simulink library "BTM_lib"  (Simulink 7.4)
settings: Solver=ode45  StartTime=0.0  StopTime=10.0  RelTol=1e-3
values from neighbouring files (symbols this model uses):
  BTMc_t_AirOutMaxTemp_fault = mpt.Parameter    [BTM_CAL.m]
  BTMc_t_AirOutMaxTemp_warn = mpt.Parameter    [BTM_CAL.m]
  BTMc_t_BCUTempOver_fatal = mpt.Parameter    [BTM_CAL.m]
  BTMc_t_BCUTempOver_fault = mpt.Parameter    [BTM_CAL.m]
  BTMc_t_BCUTempOver_warn = mpt.Parameter    [BTM_CAL.m]
  BTMc_t_BMUTempOver_fatal = mpt.Parameter    [BTM_CAL.m]
  BTMc_t_BMUTempOver_fault = mpt.Parameter    [BTM_CAL.m]
  BTMc_t_BMUTempOver_warn = mpt.Parameter    [BTM_CAL.m]
  BTMc_t_MdlTempDifOver_fatal = mpt.Parameter    [BTM_CAL.m]
  BTMc_t_MdlTempDifOver_fault = mpt.Parameter    [BTM_CAL.m]
  BTMc_t_MdlTempDifOver_warn = mpt.Parameter    [BTM_CAL.m]
  BTMc_t_MdlTempOver_fatal = mpt.Parameter    [BTM_CAL.m]
  BTMc_t_MdlTempOver_fault = mpt.Parameter    [BTM_CAL.m]
  BTMc_t_MdlTempOver_warn = mpt.Parameter    [BTM_CAL.m]
  BTMc_t_MdlTempUnder_fatal = mpt.Parameter    [BTM_CAL.m]
  BTMc_t_MdlTempUnder_fault = mpt.Parameter    [BTM_CAL.m]
  BTMc_t_MdlTempUnder_warn = mpt.Parameter    [BTM_CAL.m]
undefined symbols (not defined in the file or in its folder): PACK_Const_MdlNumOfPack, PACK_Const_TempSnrNumOfMdl
settings Model: Creator=zhangyunyun  LastModifiedBy=sunsijun

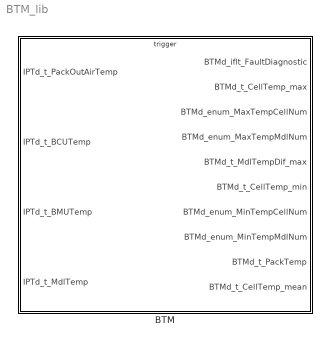
== system BTM_lib ==
  BTM : Subsystem  TreatAsAtomicUnit=on

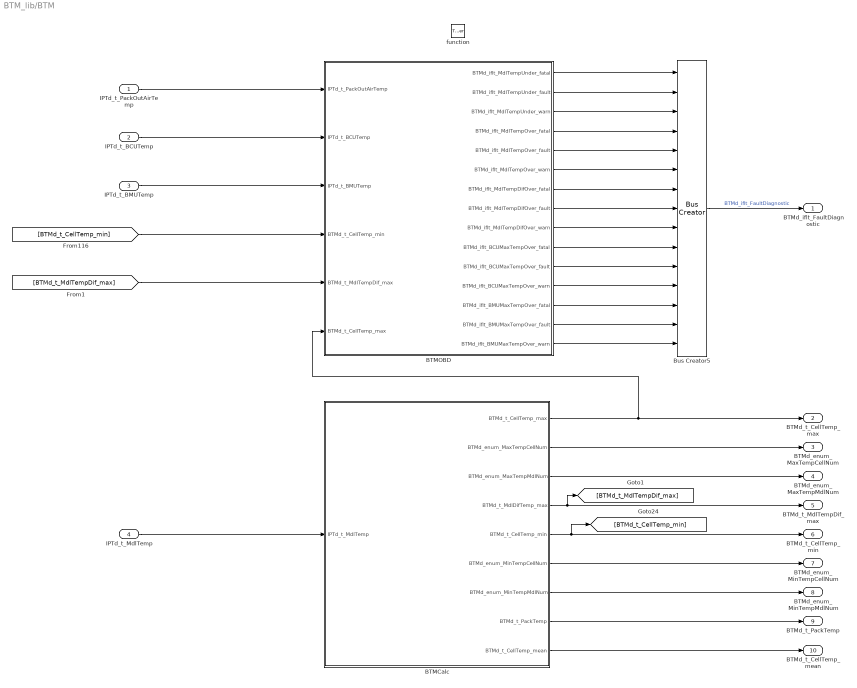
== system BTM_lib/BTM ==
  IPTd_t_PackOutAirTemp : Inport
  IPTd_t_BCUTemp : Inport  Port=2
  IPTd_t_BMUTemp : Inport  Port=3
  IPTd_t_MdlTemp : Inport  Port=4  DataType=single  OutDataTypeStr=single
  function : TriggerPort  TriggerType=function-call
  BTMCalc : Subsystem
  BTMOBD : Subsystem
  Bus Creator5 : BusCreator  Inputs=15
  BTMd_iflt_FaultDiagnostic : Outport  OutDataType=fixdt(1, 16)  OutScaling=2^0
  BTMd_t_CellTemp_max : Outport  Port=2  OutDataType=fixdt(1, 16)  OutScaling=2^0
  BTMd_enum_MaxTempCellNum : Outport  Port=3  OutDataType=fixdt(1, 16)  OutScaling=2^0
  BTMd_enum_MaxTempMdlNum : Outport  Port=4  OutDataType=fixdt(1, 16)  OutScaling=2^0
  BTMd_t_MdlTempDif_max : Outport  Port=5  OutDataType=fixdt(1, 16)  OutScaling=2^0
  BTMd_t_CellTemp_min : Outport  Port=6  OutDataType=fixdt(1, 16)  OutScaling=2^0
  BTMd_enum_MinTempCellNum : Outport  Port=7  OutDataType=fixdt(1, 16)  OutScaling=2^0
  BTMd_enum_MinTempMdlNum : Outport  Port=8  OutDataType=fixdt(1, 16)  OutScaling=2^0
  BTMd_t_PackTemp : Outport  Port=9  OutDataType=fixdt(1, 16)  OutScaling=2^0
  BTMd_t_CellTemp_mean : Outport  Port=10  OutDataType=fixdt(1, 16)  OutScaling=2^0
  wires:
  [BTMd_t_MdlTempDif_max] -> BTMOBD/5(BTMd_t_MdlTempDif_max)
  [BTMd_t_CellTemp_min] -> BTMOBD/4(BTMd_t_CellTemp_min)
  IPTd_t_BMUTemp/1 -> BTMOBD/3(IPTd_t_BMUTemp)
  BTMCalc/7(BTMd_enum_MinTempMdlNum) -> BTMd_enum_MinTempMdlNum/1
  BTMCalc/9(BTMd_t_CellTemp_mean) -> BTMd_t_CellTemp_mean/1
  BTMCalc/3(BTMd_enum_MaxTempMdlNum) -> BTMd_enum_MaxTempMdlNum/1
  IPTd_t_BCUTemp/1 -> BTMOBD/2(IPTd_t_BCUTemp)
  IPTd_t_PackOutAirTemp/1 -> BTMOBD/1(IPTd_t_PackOutAirTemp)
  BTMCalc/6(BTMd_enum_MinTempCellNum) -> BTMd_enum_MinTempCellNum/1
  IPTd_t_MdlTemp/1 -> BTMCalc/1(IPTd_t_MdlTemp)
  BTMCalc/4(BTMd_t_MdlDifTemp_max) -> [BTMd_t_MdlTempDif_max], BTMd_t_MdlTempDif_max/1
  BTMCalc/5(BTMd_t_CellTemp_min) -> [BTMd_t_CellTemp_min], BTMd_t_CellTemp_min/1
  BTMCalc/8(BTMd_t_PackTemp) -> BTMd_t_PackTemp/1
  BTMCalc/2(BTMd_enum_MaxTempCellNum) -> BTMd_enum_MaxTempCellNum/1
  BTMCalc/1(BTMd_t_CellTemp_max) -> BTMOBD/6(BTMd_t_CellTemp_max), BTMd_t_CellTemp_max/1
  BTMOBD/1(BTMd_iflt_MdlTempUnder_fatal) -> Bus Creator5/1
  BTMOBD/2(BTMd_iflt_MdlTempUnder_fault) -> Bus Creator5/2
  BTMOBD/3(BTMd_iflt_MdlTempUnder_warn) -> Bus Creator5/3
  BTMOBD/4(BTMd_iflt_MdlTempOver_fatal) -> Bus Creator5/4
  BTMOBD/5(BTMd_iflt_MdlTempOver_fault) -> Bus Creator5/5
  BTMOBD/6(BTMd_iflt_MdlTempOver_warn) -> Bus Creator5/6
  BTMOBD/7(BTMd_iflt_MdlTempDifOver_fatal) -> Bus Creator5/7
  BTMOBD/8(BTMd_iflt_MdlTempDifOver_fault) -> Bus Creator5/8
  BTMOBD/9(BTMd_iflt_MdlTempDifOver_warn) -> Bus Creator5/9
  BTMOBD/10(BTMd_iflt_BCUMaxTempOver_fatal) -> Bus Creator5/10
  BTMOBD/11(BTMd_iflt_BCUMaxTempOver_fault) -> Bus Creator5/11
  BTMOBD/12(BTMd_iflt_BCUMaxTempOver_warn) -> Bus Creator5/12
  BTMOBD/13(BTMd_iflt_BMUMaxTempOver_fatal) -> Bus Creator5/13
  BTMOBD/14(BTMd_iflt_BMUMaxTempOver_fault) -> Bus Creator5/14
  BTMOBD/15(BTMd_iflt_BMUMaxTempOver_warn) -> Bus Creator5/15
  Bus Creator5/1 -> BTMd_iflt_FaultDiagnostic/1  "BTMd_iflt_FaultDiagnostic"

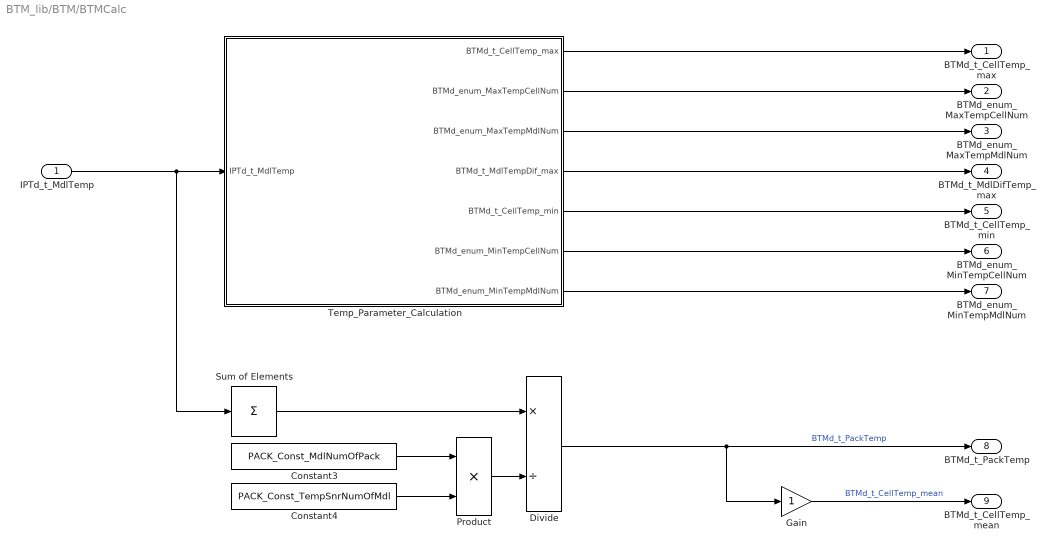
== system BTM_lib/BTM/BTMCalc ==
  IPTd_t_MdlTemp : Inport
  Constant3 : Constant  Value=PACK_Const_MdlNumOfPack  OutDataTypeMode=uint16  OutDataType=fixdt(1, 16)  OutScaling=2^0  OutDataTypeStr=uint16
  Constant4 : Constant  Value=PACK_Const_TempSnrNumOfMdl  OutDataTypeMode=uint16  OutDataType=fixdt(1, 16)  OutScaling=2^0  OutDataTypeStr=uint16
  Divide : Product  Inputs=*/  OutDataType=fixdt(1, 16)  OutScaling=2^-10
  Gain : Gain  ParameterDataType=fixdt(1, 16)  ParameterScaling=2^0  OutDataType=fixdt(1, 16)  OutScaling=2^0
  Product : Product  OutDataType=fixdt(1, 16)  OutScaling=2^0  RndMeth=Zero
  Sum of Elements : Sum  Inputs=+  OutDataType=fixdt(1, 16)  OutScaling=2^-10
  Temp_Parameter_Calculation : Subsystem  TreatAsAtomicUnit=on
  BTMd_t_CellTemp_max : Outport  OutDataType=fixdt(1, 16)  OutScaling=2^0
  BTMd_enum_MaxTempCellNum : Outport  Port=2  OutDataType=fixdt(1, 16)  OutScaling=2^0
  BTMd_enum_MaxTempMdlNum : Outport  Port=3  OutDataType=fixdt(1, 16)  OutScaling=2^0
  BTMd_t_MdlDifTemp_max : Outport  Port=4  OutDataType=fixdt(1, 16)  OutScaling=2^0
  BTMd_t_CellTemp_min : Outport  Port=5  OutDataType=fixdt(1, 16)  OutScaling=2^0
  BTMd_enum_MinTempCellNum : Outport  Port=6  OutDataType=fixdt(1, 16)  OutScaling=2^0
  BTMd_enum_MinTempMdlNum : Outport  Port=7  OutDataType=fixdt(1, 16)  OutScaling=2^0
  BTMd_t_PackTemp : Outport  Port=8
  BTMd_t_CellTemp_mean : Outport  Port=9  OutDataType=fixdt(1, 16)  OutScaling=2^0
  wires:
  Temp_Parameter_Calculation/7(BTMd_enum_MinTempMdlNum) -> BTMd_enum_MinTempMdlNum/1
  Gain/1 -> BTMd_t_CellTemp_mean/1  "BTMd_t_CellTemp_mean"
  Temp_Parameter_Calculation/3(BTMd_enum_MaxTempMdlNum) -> BTMd_enum_MaxTempMdlNum/1
  Temp_Parameter_Calculation/6(BTMd_enum_MinTempCellNum) -> BTMd_enum_MinTempCellNum/1
  Product/1 -> Divide/2
  Sum of Elements/1 -> Divide/1
  Temp_Parameter_Calculation/4(BTMd_t_MdlTempDif_max) -> BTMd_t_MdlDifTemp_max/1
  Temp_Parameter_Calculation/5(BTMd_t_CellTemp_min) -> BTMd_t_CellTemp_min/1
  Temp_Parameter_Calculation/1(BTMd_t_CellTemp_max) -> BTMd_t_CellTemp_max/1
  Divide/1 -> Gain/1, BTMd_t_PackTemp/1  "BTMd_t_PackTemp"
  IPTd_t_MdlTemp/1 -> Sum of Elements/1, Temp_Parameter_Calculation/1(IPTd_t_MdlTemp)
  Temp_Parameter_Calculation/2(BTMd_enum_MaxTempCellNum) -> BTMd_enum_MaxTempCellNum/1
  Constant3/1 -> Product/1
  Constant4/1 -> Product/2

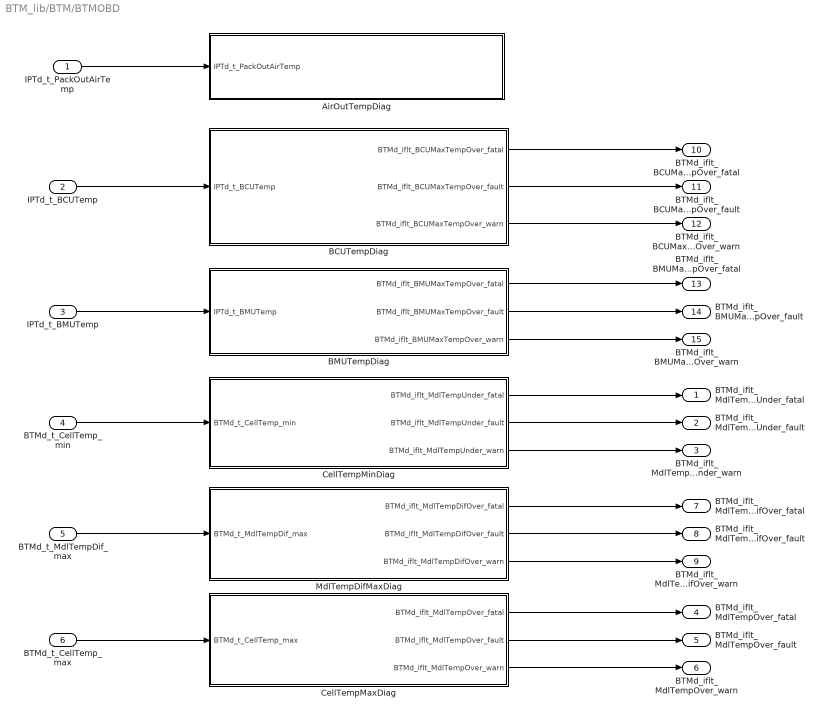
== system BTM_lib/BTM/BTMOBD ==
  IPTd_t_PackOutAirTemp : Inport
  IPTd_t_BCUTemp : Inport  Port=2
  IPTd_t_BMUTemp : Inport  Port=3
  BTMd_t_CellTemp_min : Inport  Port=4  OutDataType=fixdt(1, 16)  OutScaling=2^0
  BTMd_t_MdlTempDif_max : Inport  Port=5  OutDataType=fixdt(1, 16)  OutScaling=2^0
  BTMd_t_CellTemp_max : Inport  Port=6  OutDataType=fixdt(1, 16)  OutScaling=2^0
  AirOutTempDiag : Subsystem  TreatAsAtomicUnit=on
  BCUTempDiag : Subsystem  TreatAsAtomicUnit=on
  BMUTempDiag : Subsystem  TreatAsAtomicUnit=on
  CellTempMaxDiag : Subsystem  TreatAsAtomicUnit=on
  CellTempMinDiag : Subsystem  TreatAsAtomicUnit=on
  MdlTempDifMaxDiag : Subsystem  TreatAsAtomicUnit=on
  BTMd_iflt_MdlTempUnder_fatal : Outport  OutDataType=fixdt(1, 16)  OutScaling=2^0
  BTMd_iflt_MdlTempUnder_fault : Outport  Port=2  OutDataType=fixdt(1, 16)  OutScaling=2^0
  BTMd_iflt_MdlTempUnder_warn : Outport  Port=3  OutDataType=fixdt(1, 16)  OutScaling=2^0
  BTMd_iflt_MdlTempOver_fatal : Outport  Port=4  OutDataType=fixdt(1, 16)  OutScaling=2^0
  BTMd_iflt_MdlTempOver_fault : Outport  Port=5  OutDataType=fixdt(1, 16)  OutScaling=2^0
  BTMd_iflt_MdlTempOver_warn : Outport  Port=6  OutDataType=fixdt(1, 16)  OutScaling=2^0
  BTMd_iflt_MdlTempDifOver_fatal : Outport  Port=7  OutDataType=fixdt(1, 16)  OutScaling=2^0
  BTMd_iflt_MdlTempDifOver_fault : Outport  Port=8  OutDataType=fixdt(1, 16)  OutScaling=2^0
  BTMd_iflt_MdlTempDifOver_warn : Outport  Port=9  OutDataType=fixdt(1, 16)  OutScaling=2^0
  BTMd_iflt_BCUMaxTempOver_fatal : Outport  Port=10  OutDataType=fixdt(1, 16)  OutScaling=2^0
  BTMd_iflt_BCUMaxTempOver_fault : Outport  Port=11  OutDataType=fixdt(1, 16)  OutScaling=2^0
  BTMd_iflt_BCUMaxTempOver_warn : Outport  Port=12  OutDataType=fixdt(1, 16)  OutScaling=2^0
  BTMd_iflt_BMUMaxTempOver_fatal : Outport  Port=13  OutDataType=fixdt(1, 16)  OutScaling=2^0
  BTMd_iflt_BMUMaxTempOver_fault : Outport  Port=14  OutDataType=fixdt(1, 16)  OutScaling=2^0
  BTMd_iflt_BMUMaxTempOver_warn : Outport  Port=15  OutDataType=fixdt(1, 16)  OutScaling=2^0
  wires:
  MdlTempDifMaxDiag/3(BTMd_iflt_MdlTempDifOver_warn) -> BTMd_iflt_MdlTempDifOver_warn/1
  MdlTempDifMaxDiag/2(BTMd_iflt_MdlTempDifOver_fault) -> BTMd_iflt_MdlTempDifOver_fault/1
  MdlTempDifMaxDiag/1(BTMd_iflt_MdlTempDifOver_fatal) -> BTMd_iflt_MdlTempDifOver_fatal/1
  BTMd_t_MdlTempDif_max/1 -> MdlTempDifMaxDiag/1(BTMd_t_MdlTempDif_max)
  CellTempMaxDiag/3(BTMd_iflt_MdlTempOver_warn) -> BTMd_iflt_MdlTempOver_warn/1
  CellTempMaxDiag/2(BTMd_iflt_MdlTempOver_fault) -> BTMd_iflt_MdlTempOver_fault/1
  CellTempMaxDiag/1(BTMd_iflt_MdlTempOver_fatal) -> BTMd_iflt_MdlTempOver_fatal/1
  BTMd_t_CellTemp_max/1 -> CellTempMaxDiag/1(BTMd_t_CellTemp_max)
  CellTempMinDiag/3(BTMd_iflt_MdlTempUnder_warn) -> BTMd_iflt_MdlTempUnder_warn/1
  CellTempMinDiag/2(BTMd_iflt_MdlTempUnder_fault) -> BTMd_iflt_MdlTempUnder_fault/1
  CellTempMinDiag/1(BTMd_iflt_MdlTempUnder_fatal) -> BTMd_iflt_MdlTempUnder_fatal/1
  BTMd_t_CellTemp_min/1 -> CellTempMinDiag/1(BTMd_t_CellTemp_min)
  BMUTempDiag/3(BTMd_iflt_BMUMaxTempOver_warn) -> BTMd_iflt_BMUMaxTempOver_warn/1
  BMUTempDiag/2(BTMd_iflt_BMUMaxTempOver_fault) -> BTMd_iflt_BMUMaxTempOver_fault/1
  BMUTempDiag/1(BTMd_iflt_BMUMaxTempOver_fatal) -> BTMd_iflt_BMUMaxTempOver_fatal/1
  IPTd_t_BMUTemp/1 -> BMUTempDiag/1(IPTd_t_BMUTemp)
  BCUTempDiag/3(BTMd_iflt_BCUMaxTempOver_warn) -> BTMd_iflt_BCUMaxTempOver_warn/1
  BCUTempDiag/2(BTMd_iflt_BCUMaxTempOver_fault) -> BTMd_iflt_BCUMaxTempOver_fault/1
  BCUTempDiag/1(BTMd_iflt_BCUMaxTempOver_fatal) -> BTMd_iflt_BCUMaxTempOver_fatal/1
  IPTd_t_BCUTemp/1 -> BCUTempDiag/1(IPTd_t_BCUTemp)
  IPTd_t_PackOutAirTemp/1 -> AirOutTempDiag/1(IPTd_t_PackOutAirTemp)

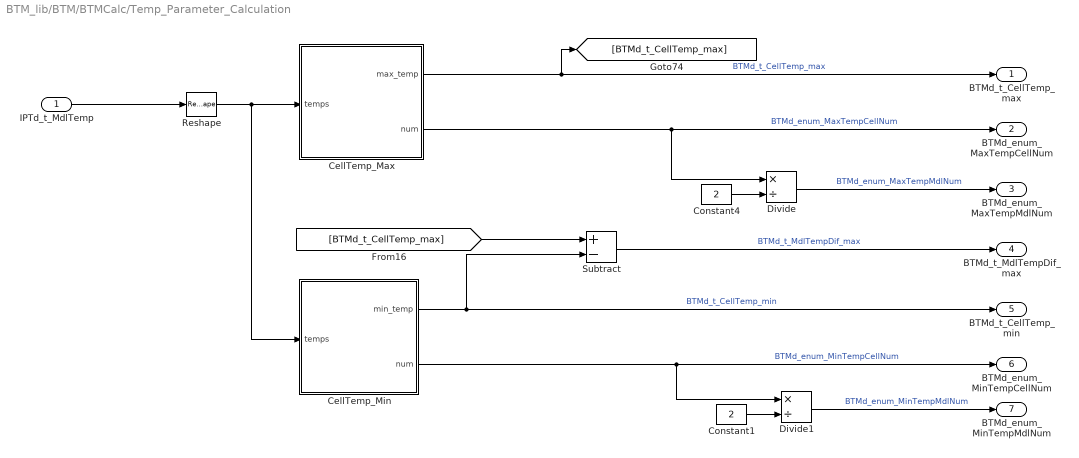
== system BTM_lib/BTM/BTMCalc/Temp_Parameter_Calculation ==
  IPTd_t_MdlTemp : Inport  OutDataType=fixdt(1, 16)  OutScaling=2^0
  CellTemp_Max : Stateflow chart
  CellTemp_Min : Stateflow chart
  Constant1 : Constant  Value=2  OutDataTypeMode=uint8  OutDataType=fixdt(1, 16)  OutScaling=2^0  OutDataTypeStr=uint8
  Constant4 : Constant  Value=2  OutDataTypeMode=uint8  OutDataType=fixdt(1, 16)  OutScaling=2^0  OutDataTypeStr=uint8
  Divide : Product  Inputs=*/  OutDataTypeMode=uint8  OutDataType=fixdt(1, 16)  OutScaling=2^-10  OutDataTypeStr=uint8  RndMeth=Ceiling
  Divide1 : Product  Inputs=*/  OutDataTypeMode=uint8  OutDataType=fixdt(1, 16)  OutScaling=2^-10  OutDataTypeStr=uint8  RndMeth=Ceiling
  Reshape : Reshape
  Subtract : Sum  Inputs=+-  OutDataType=fixdt(1, 16)  OutScaling=2^-10
  BTMd_t_CellTemp_max : Outport  OutDataType=fixdt(1, 16)  OutScaling=2^0
  BTMd_enum_MaxTempCellNum : Outport  Port=2  OutDataType=fixdt(1, 16)  OutScaling=2^0
  BTMd_enum_MaxTempMdlNum : Outport  Port=3  OutDataType=fixdt(1, 16)  OutScaling=2^0
  BTMd_t_MdlTempDif_max : Outport  Port=4  OutDataType=fixdt(1, 16)  OutScaling=2^0
  BTMd_t_CellTemp_min : Outport  Port=5  OutDataType=fixdt(1, 16)  OutScaling=2^0
  BTMd_enum_MinTempCellNum : Outport  Port=6  OutDataType=fixdt(1, 16)  OutScaling=2^0
  BTMd_enum_MinTempMdlNum : Outport  Port=7  OutDataType=fixdt(1, 16)  OutScaling=2^0
  wires:
  [BTMd_t_CellTemp_max] -> Subtract/1
  Divide1/1 -> BTMd_enum_MinTempMdlNum/1  "BTMd_enum_MinTempMdlNum"
  Constant1/1 -> Divide1/2
  Divide/1 -> BTMd_enum_MaxTempMdlNum/1  "BTMd_enum_MaxTempMdlNum"
  Constant4/1 -> Divide/2
  CellTemp_Min/2(num) -> Divide1/1, BTMd_enum_MinTempCellNum/1  "BTMd_enum_MinTempCellNum"
  Subtract/1 -> BTMd_t_MdlTempDif_max/1  "BTMd_t_MdlTempDif_max"
  CellTemp_Min/1(min_temp) -> Subtract/2, BTMd_t_CellTemp_min/1  "BTMd_t_CellTemp_min"
  Reshape/1 -> CellTemp_Min/1(temps), CellTemp_Max/1(temps)
  IPTd_t_MdlTemp/1 -> Reshape/1
  CellTemp_Max/2(num) -> Divide/1, BTMd_enum_MaxTempCellNum/1  "BTMd_enum_MaxTempCellNum"
  CellTemp_Max/1(max_temp) -> BTMd_t_CellTemp_max/1, [BTMd_t_CellTemp_max]  "BTMd_t_CellTemp_max"

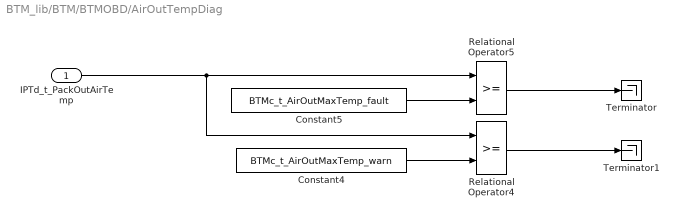
== system BTM_lib/BTM/BTMOBD/AirOutTempDiag ==
  IPTd_t_PackOutAirTemp : Inport
  Constant4 : Constant  Value=BTMc_t_AirOutMaxTemp_warn  OutDataType=fixdt(1, 16)  OutScaling=2^0
  Constant5 : Constant  Value=BTMc_t_AirOutMaxTemp_fault  OutDataType=fixdt(1, 16)  OutScaling=2^0
  Relational Operator4 : RelationalOperator  LogicOutDataTypeMode=boolean  LogicDataType=fixdt(0, 8)  OutDataTypeStr=boolean
  Relational Operator5 : RelationalOperator  LogicOutDataTypeMode=boolean  LogicDataType=fixdt(0, 8)  OutDataTypeStr=boolean
  Terminator : Terminator
  Terminator1 : Terminator
  wires:
  IPTd_t_PackOutAirTemp/1 -> Relational Operator5/1, Relational Operator4/1
  Constant5/1 -> Relational Operator5/2
  Constant4/1 -> Relational Operator4/2
  Relational Operator4/1 -> Terminator1/1
  Relational Operator5/1 -> Terminator/1

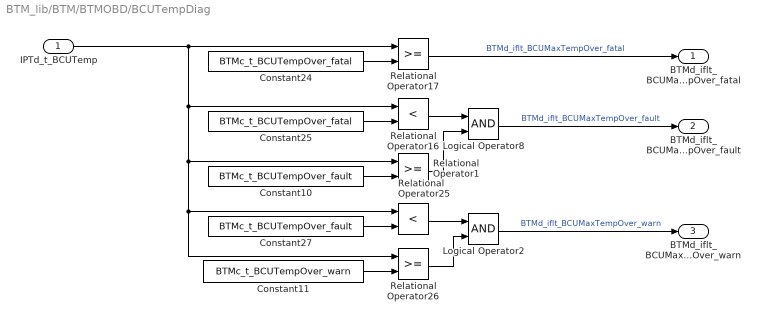
== system BTM_lib/BTM/BTMOBD/BCUTempDiag ==
  IPTd_t_BCUTemp : Inport
  Constant10 : Constant  Value=BTMc_t_BCUTempOver_fault  OutDataType=fixdt(1, 16)  OutScaling=2^0
  Constant11 : Constant  Value=BTMc_t_BCUTempOver_warn  OutDataType=fixdt(1, 16)  OutScaling=2^0
  Constant24 : Constant  Value=BTMc_t_BCUTempOver_fatal  OutDataType=fixdt(1, 16)  OutScaling=2^0
  Constant25 : Constant  Value=BTMc_t_BCUTempOver_fatal  OutDataType=fixdt(1, 16)  OutScaling=2^0
  Constant27 : Constant  Value=BTMc_t_BCUTempOver_fault  OutDataType=fixdt(1, 16)  OutScaling=2^0
  Logical Operator2 : Logic  AllPortsSameDT=off  OutDataTypeMode=boolean  LogicDataType=fixdt(0, 8)  OutDataTypeStr=boolean
  Logical Operator8 : Logic  AllPortsSameDT=off  OutDataTypeMode=boolean  LogicDataType=fixdt(0, 8)  OutDataTypeStr=boolean
  Relational Operator1 : RelationalOperator  LogicOutDataTypeMode=boolean  LogicDataType=fixdt(0, 8)  OutDataTypeStr=boolean
  Relational Operator16 : RelationalOperator  Operator=<  LogicOutDataTypeMode=boolean  LogicDataType=fixdt(0, 8)  OutDataTypeStr=boolean
  Relational Operator17 : RelationalOperator  LogicOutDataTypeMode=boolean  LogicDataType=fixdt(0, 8)  OutDataTypeStr=boolean
  Relational Operator25 : RelationalOperator  Operator=<  LogicOutDataTypeMode=boolean  LogicDataType=fixdt(0, 8)  OutDataTypeStr=boolean
  Relational Operator26 : RelationalOperator  LogicOutDataTypeMode=boolean  LogicDataType=fixdt(0, 8)  OutDataTypeStr=boolean
  BTMd_iflt_BCUMaxTempOver_fatal : Outport  OutDataType=fixdt(1, 16)  OutScaling=2^0
  BTMd_iflt_BCUMaxTempOver_fault : Outport  Port=2  OutDataType=fixdt(1, 16)  OutScaling=2^0
  BTMd_iflt_BCUMaxTempOver_warn : Outport  Port=3  OutDataType=fixdt(1, 16)  OutScaling=2^0
  wires:
  IPTd_t_BCUTemp/1 -> Relational Operator26/1, Relational Operator25/1, Relational Operator1/1, Relational Operator16/1, Relational Operator17/1
  Constant24/1 -> Relational Operator17/2
  Constant27/1 -> Relational Operator25/2
  Constant10/1 -> Relational Operator1/2
  Constant25/1 -> Relational Operator16/2
  Relational Operator26/1 -> Logical Operator2/2
  Relational Operator17/1 -> BTMd_iflt_BCUMaxTempOver_fatal/1  "BTMd_iflt_BCUMaxTempOver_fatal"
  Logical Operator8/1 -> BTMd_iflt_BCUMaxTempOver_fault/1  "BTMd_iflt_BCUMaxTempOver_fault"
  Relational Operator1/1 -> Logical Operator8/2
  Relational Operator16/1 -> Logical Operator8/1
  Logical Operator2/1 -> BTMd_iflt_BCUMaxTempOver_warn/1  "BTMd_iflt_BCUMaxTempOver_warn"
  Relational Operator25/1 -> Logical Operator2/1
  Constant11/1 -> Relational Operator26/2

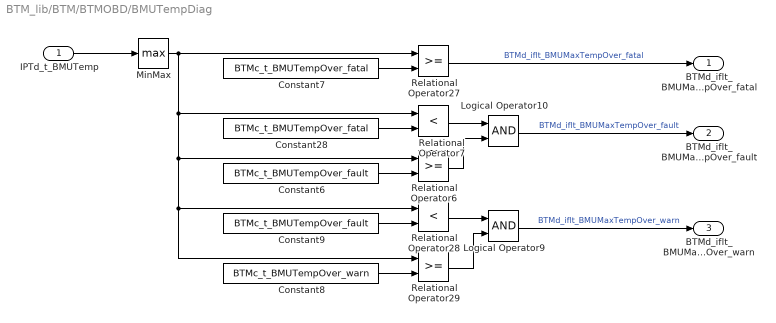
== system BTM_lib/BTM/BTMOBD/BMUTempDiag ==
  IPTd_t_BMUTemp : Inport
  Constant28 : Constant  Value=BTMc_t_BMUTempOver_fatal  OutDataType=fixdt(1, 16)  OutScaling=2^0
  Constant6 : Constant  Value=BTMc_t_BMUTempOver_fault  OutDataType=fixdt(1, 16)  OutScaling=2^0
  Constant7 : Constant  Value=BTMc_t_BMUTempOver_fatal  OutDataType=fixdt(1, 16)  OutScaling=2^0
  Constant8 : Constant  Value=BTMc_t_BMUTempOver_warn  OutDataType=fixdt(1, 16)  OutScaling=2^0
  Constant9 : Constant  Value=BTMc_t_BMUTempOver_fault  OutDataType=fixdt(1, 16)  OutScaling=2^0
  Logical Operator10 : Logic  AllPortsSameDT=off  OutDataTypeMode=boolean  LogicDataType=fixdt(0, 8)  OutDataTypeStr=boolean
  Logical Operator9 : Logic  AllPortsSameDT=off  OutDataTypeMode=boolean  LogicDataType=fixdt(0, 8)  OutDataTypeStr=boolean
  MinMax : MinMax  Function=max  OutDataType=fixdt(1, 16)  OutScaling=2^0
  Relational Operator27 : RelationalOperator  LogicOutDataTypeMode=boolean  LogicDataType=fixdt(0, 8)  OutDataTypeStr=boolean
  Relational Operator28 : RelationalOperator  Operator=<  LogicOutDataTypeMode=boolean  LogicDataType=fixdt(0, 8)  OutDataTypeStr=boolean
  Relational Operator29 : RelationalOperator  LogicOutDataTypeMode=boolean  LogicDataType=fixdt(0, 8)  OutDataTypeStr=boolean
  Relational Operator6 : RelationalOperator  LogicOutDataTypeMode=boolean  LogicDataType=fixdt(0, 8)  OutDataTypeStr=boolean
  Relational Operator7 : RelationalOperator  Operator=<  LogicOutDataTypeMode=boolean  LogicDataType=fixdt(0, 8)  OutDataTypeStr=boolean
  BTMd_iflt_BMUMaxTempOver_fatal : Outport  OutDataType=fixdt(1, 16)  OutScaling=2^0
  BTMd_iflt_BMUMaxTempOver_fault : Outport  Port=2  OutDataType=fixdt(1, 16)  OutScaling=2^0
  BTMd_iflt_BMUMaxTempOver_warn : Outport  Port=3  OutDataType=fixdt(1, 16)  OutScaling=2^0
  wires:
  MinMax/1 -> Relational Operator29/1, Relational Operator28/1, Relational Operator6/1, Relational Operator7/1, Relational Operator27/1
  IPTd_t_BMUTemp/1 -> MinMax/1
  Constant7/1 -> Relational Operator27/2
  Constant9/1 -> Relational Operator28/2
  Constant6/1 -> Relational Operator6/2
  Constant28/1 -> Relational Operator7/2
  Relational Operator29/1 -> Logical Operator9/2
  Relational Operator27/1 -> BTMd_iflt_BMUMaxTempOver_fatal/1  "BTMd_iflt_BMUMaxTempOver_fatal"
  Logical Operator10/1 -> BTMd_iflt_BMUMaxTempOver_fault/1  "BTMd_iflt_BMUMaxTempOver_fault"
  Relational Operator6/1 -> Logical Operator10/2
  Relational Operator7/1 -> Logical Operator10/1
  Logical Operator9/1 -> BTMd_iflt_BMUMaxTempOver_warn/1  "BTMd_iflt_BMUMaxTempOver_warn"
  Relational Operator28/1 -> Logical Operator9/1
  Constant8/1 -> Relational Operator29/2

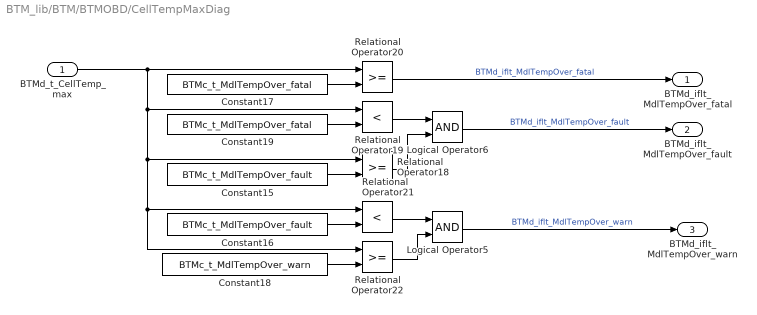
== system BTM_lib/BTM/BTMOBD/CellTempMaxDiag ==
  BTMd_t_CellTemp_max : Inport  OutDataType=fixdt(1, 16)  OutScaling=2^0
  Constant15 : Constant  Value=BTMc_t_MdlTempOver_fault  OutDataType=fixdt(1, 16)  OutScaling=2^0
  Constant16 : Constant  Value=BTMc_t_MdlTempOver_fault  OutDataType=fixdt(1, 16)  OutScaling=2^0
  Constant17 : Constant  Value=BTMc_t_MdlTempOver_fatal  OutDataType=fixdt(1, 16)  OutScaling=2^0
  Constant18 : Constant  Value=BTMc_t_MdlTempOver_warn  OutDataType=fixdt(1, 16)  OutScaling=2^0
  Constant19 : Constant  Value=BTMc_t_MdlTempOver_fatal  OutDataType=fixdt(1, 16)  OutScaling=2^0
  Logical Operator5 : Logic  AllPortsSameDT=off  OutDataTypeMode=boolean  LogicDataType=fixdt(0, 8)  OutDataTypeStr=boolean
  Logical Operator6 : Logic  AllPortsSameDT=off  OutDataTypeMode=boolean  LogicDataType=fixdt(0, 8)  OutDataTypeStr=boolean
  Relational Operator18 : RelationalOperator  LogicOutDataTypeMode=boolean  LogicDataType=fixdt(0, 8)  OutDataTypeStr=boolean
  Relational Operator19 : RelationalOperator  Operator=<  LogicOutDataTypeMode=boolean  LogicDataType=fixdt(0, 8)  OutDataTypeStr=boolean
  Relational Operator20 : RelationalOperator  LogicOutDataTypeMode=boolean  LogicDataType=fixdt(0, 8)  OutDataTypeStr=boolean
  Relational Operator21 : RelationalOperator  Operator=<  LogicOutDataTypeMode=boolean  LogicDataType=fixdt(0, 8)  OutDataTypeStr=boolean
  Relational Operator22 : RelationalOperator  LogicOutDataTypeMode=boolean  LogicDataType=fixdt(0, 8)  OutDataTypeStr=boolean
  BTMd_iflt_MdlTempOver_fatal : Outport  OutDataType=fixdt(1, 16)  OutScaling=2^0
  BTMd_iflt_MdlTempOver_fault : Outport  Port=2  OutDataType=fixdt(1, 16)  OutScaling=2^0
  BTMd_iflt_MdlTempOver_warn : Outport  Port=3  OutDataType=fixdt(1, 16)  OutScaling=2^0
  wires:
  BTMd_t_CellTemp_max/1 -> Relational Operator22/1, Relational Operator21/1, Relational Operator18/1, Relational Operator19/1, Relational Operator20/1
  Constant17/1 -> Relational Operator20/2
  Constant16/1 -> Relational Operator21/2
  Constant15/1 -> Relational Operator18/2
  Constant19/1 -> Relational Operator19/2
  Relational Operator22/1 -> Logical Operator5/2
  Relational Operator20/1 -> BTMd_iflt_MdlTempOver_fatal/1  "BTMd_iflt_MdlTempOver_fatal"
  Logical Operator6/1 -> BTMd_iflt_MdlTempOver_fault/1  "BTMd_iflt_MdlTempOver_fault"
  Relational Operator18/1 -> Logical Operator6/2
  Relational Operator19/1 -> Logical Operator6/1
  Logical Operator5/1 -> BTMd_iflt_MdlTempOver_warn/1  "BTMd_iflt_MdlTempOver_warn"
  Relational Operator21/1 -> Logical Operator5/1
  Constant18/1 -> Relational Operator22/2

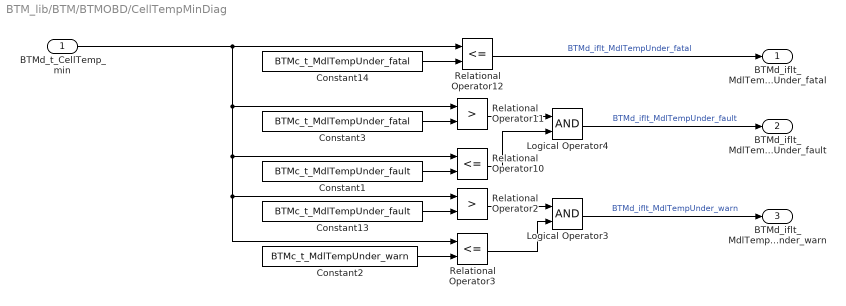
== system BTM_lib/BTM/BTMOBD/CellTempMinDiag ==
  BTMd_t_CellTemp_min : Inport  OutDataType=fixdt(1, 16)  OutScaling=2^0
  Constant1 : Constant  Value=BTMc_t_MdlTempUnder_fault  OutDataType=fixdt(1, 16)  OutScaling=2^0
  Constant13 : Constant  Value=BTMc_t_MdlTempUnder_fault  OutDataType=fixdt(1, 16)  OutScaling=2^0
  Constant14 : Constant  Value=BTMc_t_MdlTempUnder_fatal  OutDataType=fixdt(1, 16)  OutScaling=2^0
  Constant2 : Constant  Value=BTMc_t_MdlTempUnder_warn  OutDataType=fixdt(1, 16)  OutScaling=2^0
  Constant3 : Constant  Value=BTMc_t_MdlTempUnder_fatal  OutDataType=fixdt(1, 16)  OutScaling=2^0
  Logical Operator3 : Logic  AllPortsSameDT=off  OutDataTypeMode=boolean  LogicDataType=fixdt(0, 8)  OutDataTypeStr=boolean
  Logical Operator4 : Logic  AllPortsSameDT=off  OutDataTypeMode=boolean  LogicDataType=fixdt(0, 8)  OutDataTypeStr=boolean
  Relational Operator10 : RelationalOperator  Operator=<=  LogicOutDataTypeMode=boolean  LogicDataType=fixdt(0, 8)  OutDataTypeStr=boolean
  Relational Operator11 : RelationalOperator  Operator=>  LogicOutDataTypeMode=boolean  LogicDataType=fixdt(0, 8)  OutDataTypeStr=boolean
  Relational Operator12 : RelationalOperator  Operator=<=  LogicOutDataTypeMode=boolean  LogicDataType=fixdt(0, 8)  OutDataTypeStr=boolean
  Relational Operator2 : RelationalOperator  Operator=>  LogicOutDataTypeMode=boolean  LogicDataType=fixdt(0, 8)  OutDataTypeStr=boolean
  Relational Operator3 : RelationalOperator  Operator=<=  LogicOutDataTypeMode=boolean  LogicDataType=fixdt(0, 8)  OutDataTypeStr=boolean
  BTMd_iflt_MdlTempUnder_fatal : Outport  OutDataType=fixdt(1, 16)  OutScaling=2^0
  BTMd_iflt_MdlTempUnder_fault : Outport  Port=2  OutDataType=fixdt(1, 16)  OutScaling=2^0
  BTMd_iflt_MdlTempUnder_warn : Outport  Port=3  OutDataType=fixdt(1, 16)  OutScaling=2^0
  wires:
  BTMd_t_CellTemp_min/1 -> Relational Operator3/1, Relational Operator2/1, Relational Operator10/1, Relational Operator11/1, Relational Operator12/1
  Constant14/1 -> Relational Operator12/2
  Constant13/1 -> Relational Operator2/2
  Constant1/1 -> Relational Operator10/2
  Constant3/1 -> Relational Operator11/2
  Relational Operator3/1 -> Logical Operator3/2
  Relational Operator12/1 -> BTMd_iflt_MdlTempUnder_fatal/1  "BTMd_iflt_MdlTempUnder_fatal"
  Logical Operator4/1 -> BTMd_iflt_MdlTempUnder_fault/1  "BTMd_iflt_MdlTempUnder_fault"
  Relational Operator10/1 -> Logical Operator4/2
  Relational Operator11/1 -> Logical Operator4/1
  Logical Operator3/1 -> BTMd_iflt_MdlTempUnder_warn/1  "BTMd_iflt_MdlTempUnder_warn"
  Relational Operator2/1 -> Logical Operator3/1
  Constant2/1 -> Relational Operator3/2

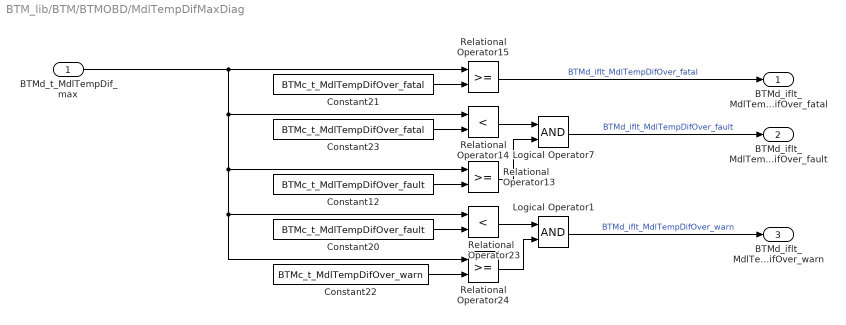
== system BTM_lib/BTM/BTMOBD/MdlTempDifMaxDiag ==
  BTMd_t_MdlTempDif_max : Inport  OutDataType=fixdt(1, 16)  OutScaling=2^0
  Constant12 : Constant  Value=BTMc_t_MdlTempDifOver_fault  OutDataType=fixdt(1, 16)  OutScaling=2^0
  Constant20 : Constant  Value=BTMc_t_MdlTempDifOver_fault  OutDataType=fixdt(1, 16)  OutScaling=2^0
  Constant21 : Constant  Value=BTMc_t_MdlTempDifOver_fatal  OutDataType=fixdt(1, 16)  OutScaling=2^0
  Constant22 : Constant  Value=BTMc_t_MdlTempDifOver_warn  OutDataType=fixdt(1, 16)  OutScaling=2^0
  Constant23 : Constant  Value=BTMc_t_MdlTempDifOver_fatal  OutDataType=fixdt(1, 16)  OutScaling=2^0
  Logical Operator1 : Logic  AllPortsSameDT=off  OutDataTypeMode=boolean  LogicDataType=fixdt(0, 8)  OutDataTypeStr=boolean
  Logical Operator7 : Logic  AllPortsSameDT=off  OutDataTypeMode=boolean  LogicDataType=fixdt(0, 8)  OutDataTypeStr=boolean
  Relational Operator13 : RelationalOperator  LogicOutDataTypeMode=boolean  LogicDataType=fixdt(0, 8)  OutDataTypeStr=boolean
  Relational Operator14 : RelationalOperator  Operator=<  LogicOutDataTypeMode=boolean  LogicDataType=fixdt(0, 8)  OutDataTypeStr=boolean
  Relational Operator15 : RelationalOperator  LogicOutDataTypeMode=boolean  LogicDataType=fixdt(0, 8)  OutDataTypeStr=boolean
  Relational Operator23 : RelationalOperator  Operator=<  LogicOutDataTypeMode=boolean  LogicDataType=fixdt(0, 8)  OutDataTypeStr=boolean
  Relational Operator24 : RelationalOperator  LogicOutDataTypeMode=boolean  LogicDataType=fixdt(0, 8)  OutDataTypeStr=boolean
  BTMd_iflt_MdlTempDifOver_fatal : Outport  OutDataType=fixdt(1, 16)  OutScaling=2^0
  BTMd_iflt_MdlTempDifOver_fault : Outport  Port=2  OutDataType=fixdt(1, 16)  OutScaling=2^0
  BTMd_iflt_MdlTempDifOver_warn : Outport  Port=3  OutDataType=fixdt(1, 16)  OutScaling=2^0
  wires:
  BTMd_t_MdlTempDif_max/1 -> Relational Operator24/1, Relational Operator23/1, Relational Operator13/1, Relational Operator14/1, Relational Operator15/1
  Constant21/1 -> Relational Operator15/2
  Constant20/1 -> Relational Operator23/2
  Constant12/1 -> Relational Operator13/2
  Constant23/1 -> Relational Operator14/2
  Relational Operator24/1 -> Logical Operator1/2
  Relational Operator15/1 -> BTMd_iflt_MdlTempDifOver_fatal/1  "BTMd_iflt_MdlTempDifOver_fatal"
  Logical Operator7/1 -> BTMd_iflt_MdlTempDifOver_fault/1  "BTMd_iflt_MdlTempDifOver_fault"
  Relational Operator13/1 -> Logical Operator7/2
  Relational Operator14/1 -> Logical Operator7/1
  Logical Operator1/1 -> BTMd_iflt_MdlTempDifOver_warn/1  "BTMd_iflt_MdlTempDifOver_warn"
  Relational Operator23/1 -> Logical Operator1/1
  Constant22/1 -> Relational Operator24/2

== matlab function BTM/BTMCalc/Temp_Parameter_Calculation/CellTemp_Min ==
  data: temps input double; min_temp output double; num output double
function [min_temp,num] = min(temps)
%#eml
[I Y]=min(temps);
min_temp = I;
num =uint8(Y);

== matlab function BTM/BTMCalc/Temp_Parameter_Calculation/CellTemp_Max ==
  data: temps input double; max_temp output double; num output double
function [max_temp,num] = max(temps)
%#eml
[I Y]=max(temps);
max_temp = I;
num =uint8(Y);
